simulink model "simulink_simulations"  (R2024a)
settings: Solver=VariableStepAuto  StartTime=0.0  StopTime=60  MaxStep=1e-2  RelTol=1e-3
values from neighbouring files (symbols this model uses):
  A = [0 1 0 0 ... (first row only)    [matlab_script.m]
  B = [0 0; 1/m 0; 0 0; 0 1/m]    [matlab_script.m]
  C = eye(4)    [matlab_script.m]
  D = zeros(4, 2)    [matlab_script.m]
  eta = 8e17    (= 8e+17)    [matlab_script.m]
  K = lqr(A, B, Q, R)    [matlab_script.m]
  K1 = 1    [matlab_script.m]
  K2 = 1    [matlab_script.m]
  m = 2e3    (= 2000)    [matlab_script.m]
  perturbation_standard_deviation = 9.6e7    (= 96000000)    [matlab_script.m]
  R_earth = 6.378e6    (= 6378000)    [matlab_script.m]
  x_eq = [r_ref; d_r_ref; theta_ref; d_theta_ref]    [matlab_script.m]
undefined symbols (not defined in the file or in its folder): Continuous, Time
libraries: ctrlSharedLib x2
settings Model: Creator=maxik  LastModifiedBy=maxik

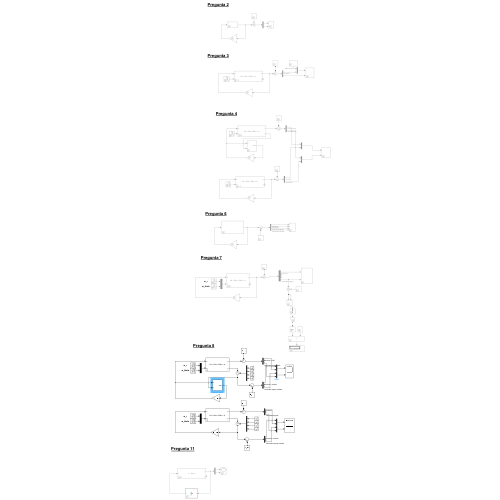
[thumbnail: Simulink's stored preview of the top-level diagram]
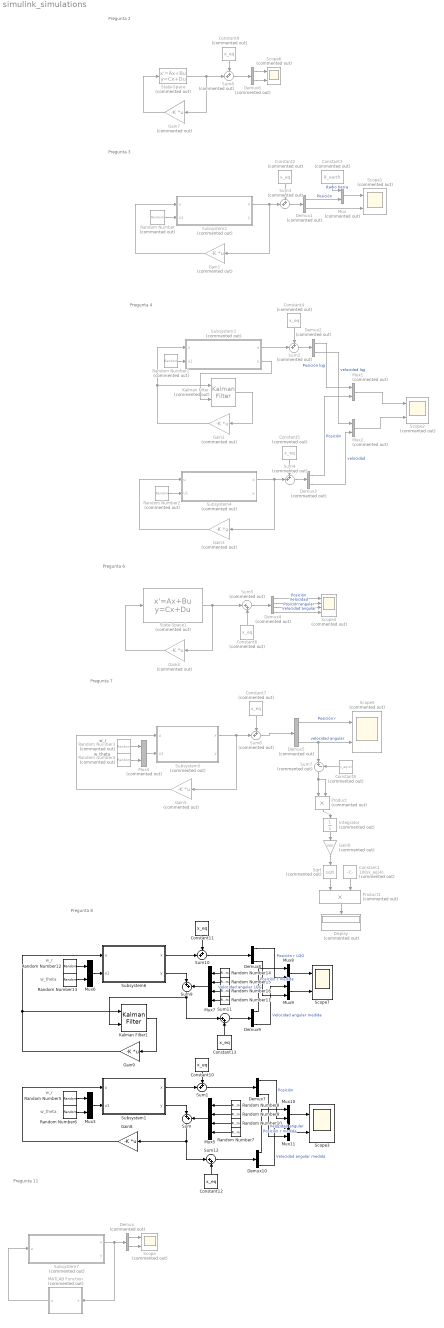
== system simulink_simulations ==
  note: Pregunta 8
  note: w_theta
  note: w_r
  note: Pregunta 2
  note: Pregunta 3
  note: Pregunta 4
  note: Pregunta 6
  note: Pregunta 7
  note: w_r
  note: w_theta
  note: w_theta
  note: w_r
  note: Pregunta 11
  Constant1 : Constant  Commented=on  Value=100/x_eq(4)
  Constant{10..13} (4 alike) : Constant  Value=x_eq
  Constant{2,4..7,9} (6 alike) : Constant  Commented=on  Value=x_eq
  Constant3 : Constant  Commented=on  Value=R_earth
  Constant8 : Constant  Commented=on  Value=x_eq(4)
  Demux{,1..3,6} (5 alike) : Demux  Commented=on  Outputs=2
  Demux{7..10} (4 alike) : Demux
  Demux4 : Demux  Commented=on
  Demux5 : Demux  Commented=on
  Display : Display  Commented=on
  Gain{1..5,7} (6 alike) : Gain  Commented=on  Gain=-K  Multiplication=Matrix(K*u) (u vector)
  Gain6 : Gain  Commented=on  Gain=1/60
  Gain8 : Gain  Gain=-K  Multiplication=Matrix(K*u) (u vector)
  Gain9 : Gain  Gain=-K  Multiplication=Matrix(K*u) (u vector)
  Integrator : Integrator  Commented=on
  Kalman Filter : ctrlSharedLib/Kalman Filter  Commented=on  TimeDomain=Continuous-Time  UseCurrentEstimator=on  ModelSource=Individual A, B, C, D matrices  ModelSourceVariable=ss(0.95,1,1,0,1)  A=A  B=B  C=C  D=D  NumberOfStates=1  NumberOfInputs=1  NumberOfOutputs=1  InitialEstimateSource=Dialog  X0=[0; 0]  P0=10  UseK=off  UseGH=on  NumberOfProcessNoiseInputs=1  G=[0; 1]  TimeInvariantG=on  H=[0; 0]  TimeInvariantH=on  Q=0 * (9.6e7)^2  TimeInvariantQ=on  R=1e-5 * eye(2)  TimeInvariantR=on  N=[0 0]  TimeInvariantN=on  AddInputPort=on  AddEnablePort=off  OutputEstimatedY=off  OutputP=off  Ts=-1
  Kalman Filter1 : ctrlSharedLib/Kalman Filter  TimeDomain=Continuous-Time  UseCurrentEstimator=on  ModelSource=Individual A, B, C, D matrices  ModelSourceVariable=ss(0.95,1,1,0,1)  A=A  B=B  C=C  D=D  NumberOfStates=1  NumberOfInputs=1  NumberOfOutputs=1  InitialEstimateSource=Dialog  X0=0  P0=10  UseK=off  UseGH=on  NumberOfProcessNoiseInputs=1  G=[0 0; 1 0; 0 0; 0 1]  TimeInvariantG=on  H=0  TimeInvariantH=on  Q="diag([(0.01*9.6e7)^2   (0.01*0.23)^2])"  TimeInvariantQ=on  R="diag([(1.6e5)^2  (1e4)^2  (1e-5)^2  (7.27e-6)^2])"  TimeInvariantR=on  N=0  TimeInvariantN=on  AddInputPort=on  AddEnablePort=off  OutputEstimatedY=off  OutputP=off  Ts=-1
  MATLAB Function : MATLAB Function  Commented=on  TreatAsAtomicUnit=on
  Mux{,1..2,4} (4 alike) : Mux  Commented=on  Inputs=2
  Mux{3,6,8..11} (6 alike) : Mux  Inputs=2
  Mux5 : Mux
  Mux7 : Mux
  Product : Product  Commented=on
  Product1 : Product  Commented=on
  Random Number : RandomNumber  Commented=on  Variance=perturbation_standard_deviation^2  Seed=25  SampleTime=1e-5
  Random Number1 : RandomNumber  Commented=on  Variance=(9.6e7)^2  Seed=25  SampleTime=1e-5
  Random Number10 : RandomNumber  Variance=(1e-5)^2  SampleTime=1e-5
  Random Number11 : RandomNumber  Variance=(7.27e-6)^2  SampleTime=1e-5
  Random Number12 : RandomNumber  Variance=(0.01 * 9.6e7)^2  Seed=25  SampleTime=1e-5
  Random Number13 : RandomNumber  Variance=(0.01 * 0.23)^2  Seed=25  SampleTime=1e-5
  Random Number14 : RandomNumber  Variance=(1.6e5)^2  SampleTime=1e-5
  Random Number15 : RandomNumber  Variance=(1e4)^2  SampleTime=1e-5
  Random Number16 : RandomNumber  Variance=(1e-5)^2  SampleTime=1e-5
  Random Number2 : RandomNumber  Commented=on  Variance=(9.6e7)^2  Seed=25  SampleTime=1e-5
  Random Number3 : RandomNumber  Commented=on  Variance=(0.01 * 9.6e7)^2  Seed=25  SampleTime=1e-5
  Random Number4 : RandomNumber  Commented=on  Variance=(0.23)^2  Seed=25  SampleTime=1e-5
  Random Number5 : RandomNumber  Variance=(0.01 * 9.6e7)^2  Seed=25  SampleTime=1e-5
  Random Number6 : RandomNumber  Variance=(0.01 * 0.23)^2  Seed=25  SampleTime=1e-5
  Random Number7 : RandomNumber  Variance=(7.27e-6)^2  SampleTime=1e-5
  Random Number8 : RandomNumber  Variance=(1.6e5)^2  SampleTime=1e-5
  Random Number9 : RandomNumber  Variance=(1e4)^2  SampleTime=1e-5
  Scope{,1..2,5..6} (5 alike) : Scope  Commented=on  NumInputPorts=2
  Scope3 : Scope  NumInputPorts=2
  Scope4 : Scope  Commented=on  NumInputPorts=4
  Scope7 : Scope  NumInputPorts=2
  Sqrt : Sqrt  Commented=on
  State-Space : StateSpace  Commented=on  A=A  B=B  C=C  D=D  InitialCondition=[1e6; -2e6]
  State-Space1 : StateSpace  Commented=on  A=A  B=B  C=C  D=D  InitialCondition=[-1e6; -1e6; 0; 0]
  Subsystem1 : Subsystem
      mask Display:
      | disp('\n\n\nΔẋ = AΔx + BΔu + w\n\n\n')
      | port_label('input', 1, 'u');
      | port_label('input', 2, 'w');
      | port_label('output', 1, 'x');
      | port_label('output', 2, 'y');
  Subsystem2 : Subsystem  Commented=on
      mask Display:
      | disp('\n\n\nΔẋ = AΔx + BΔu + w\n\n\n')
      | port_label('input', 1, 'u');
      | port_label('input', 2, 'w');
      | port_label('output', 1, 'x');
      | port_label('output', 2, 'y');
  Subsystem3 : Subsystem  Commented=on
      mask Display:
      | disp('\n\n\nΔẋ = AΔx + BΔu + w\n\n\n')
      | port_label('input', 1, 'u');
      | port_label('input', 2, 'w');
      | port_label('output', 1, 'x');
      | port_label('output', 2, 'y');
  Subsystem4 : Subsystem  Commented=on
      mask Display:
      | disp('\n\n\nΔẋ = AΔx + BΔu + w\n\n\n')
      | port_label('input', 1, 'u');
      | port_label('input', 2, 'w');
      | port_label('output', 1, 'x');
      | port_label('output', 2, 'y');
  Subsystem5 : Subsystem  Commented=on
      mask Display:
      | disp('\n\n\nΔẋ = AΔx + BΔu + w\n\n\n')
      | port_label('input', 1, 'u');
      | port_label('input', 2, 'w');
      | port_label('output', 1, 'x');
      | port_label('output', 2, 'y');
  Subsystem6 : Subsystem
      mask Display:
      | disp('\n\n\nΔẋ = AΔx + BΔu + w\n\n\n')
      | port_label('input', 1, 'u');
      | port_label('input', 2, 'w');
      | port_label('output', 1, 'x');
      | port_label('output', 2, 'y');
  Subsystem7 : Subsystem  Commented=on
      mask Display:
      | disp('\n\n\nẋ = f(x,u)\n\n\n')
      | port_label('input', 1, 'u');
      | port_label('output', 1, 'x');
      | port_label('output', 2, 'y');
  Sum{,9,11..12} (4 alike) : Sum  Inputs=|++
  Sum1 : Sum  Inputs=++|
  Sum10 : Sum  Inputs=++|
  Sum{2..4,6,8} (5 alike) : Sum  Commented=on  Inputs=++|
  Sum5 : Sum  Commented=on  Inputs=|++
  Sum7 : Sum  Commented=on  Inputs=|+-
  wires:
  Subsystem2/1(x) -> Gain1/1, Sum3/2
  Demux1/2 -> Scope1/2
  Random Number/1 -> Subsystem2/2(u1)
  Gain1/1 -> Subsystem2/1(u)
  Sum3/1 -> Demux1/1
  Constant2/1 -> Sum3/1
  Demux1/1 -> Mux/2  "Posición"
  Mux/1 -> Scope1/1
  Constant3/1 -> Mux/1  "Radio tierra"
  Gain2/1 -> Subsystem3/1(u), Kalman Filter/1
  Sum2/1 -> Demux2/1
  Subsystem3/1(x) -> Sum2/2
  Constant4/1 -> Sum2/1
  Random Number1/1 -> Subsystem3/2(u1)
  Subsystem3/2(y) -> Kalman Filter/2
  Kalman Filter/1 -> Gain2/1
  Sum4/1 -> Demux3/1
  Gain3/1 -> Subsystem4/1(u)
  Random Number2/1 -> Subsystem4/2(u1)
  Subsystem4/1(x) -> Gain3/1, Sum4/2
  Constant5/1 -> Sum4/1
  Demux2/1 -> Mux1/1  "Posición lqg"
  Demux3/1 -> Mux1/2  "Posición"
  Demux2/2 -> Mux2/1  "velocidad lqg"
  Demux3/2 -> Mux2/2  "velocidad"
  Mux2/1 -> Scope2/2
  Mux1/1 -> Scope2/1
  State-Space1/1 -> Sum5/1, Gain4/1
  Sum5/1 -> Demux4/1
  Gain4/1 -> State-Space1/1
  Constant6/1 -> Sum5/2
  Demux4/1 -> Scope4/1  "Posición"
  Demux4/4 -> Scope4/4  "Velocidad angular"
  Demux4/3 -> Scope4/3  "Posición angular"
  Demux4/2 -> Scope4/2  "Velocidad"
  Constant7/1 -> Sum6/1
  Gain5/1 -> Subsystem5/1(u)
  Subsystem5/1(x) -> Gain5/1, Sum6/2
  Sum6/1 -> Demux5/1
  Random Number3/1 -> Mux4/1
  Random Number4/1 -> Mux4/2
  Mux4/1 -> Subsystem5/2(u1)
  Demux5/1 -> Scope5/1  "Posición r"
  Demux5/4 -> Scope5/2, Sum7/1  "velocidad angular"
  Constant8/1 -> Sum7/2
  Sum7/1 -> Product/2, Product/1
  Product/1 -> Integrator/1
  Integrator/1 -> Gain6/1
  Gain6/1 -> Sqrt/1
  State-Space/1 -> Sum8/2, Gain7/1
  Gain7/1 -> State-Space/1
  Constant9/1 -> Sum8/1
  Demux6/2 -> Scope6/2
  Demux6/1 -> Scope6/1
  Sum8/1 -> Demux6/1
  Constant1/1 -> Product1/2
  Sqrt/1 -> Product1/1
  Product1/1 -> Display/1
  Mux3/1 -> Subsystem1/2(u1)
  Random Number5/1 -> Mux3/1
  Random Number6/1 -> Mux3/2
  Subsystem1/1(x) -> Sum1/2
  Constant10/1 -> Sum1/1
  Gain8/1 -> Subsystem1/1(u)
  Subsystem1/2(y) -> Sum/1
  Mux5/1 -> Sum/2
  Sum/1 -> Sum12/1, Gain8/1
  Random Number14/1 -> Mux7/1
  Random Number12/1 -> Mux6/1
  Random Number13/1 -> Mux6/2
  Mux6/1 -> Subsystem6/2(u1)
  Gain9/1 -> Subsystem6/1(u), Kalman Filter1/1
  Subsystem6/1(x) -> Sum10/2
  Random Number11/1 -> Mux7/4
  Constant11/1 -> Sum10/1
  Subsystem6/2(y) -> Sum9/1
  Mux7/1 -> Sum9/2
  Random Number15/1 -> Mux7/2
  Random Number16/1 -> Mux7/3
  Sum9/1 -> Sum11/1, Kalman Filter1/2
  Kalman Filter1/1 -> Gain9/1
  Sum1/1 -> Demux7/1
  Sum10/1 -> Demux8/1
  Subsystem7/1(x) -> Demux/1, MATLAB Function/1(x)
  MATLAB Function/1(u) -> Subsystem7/1(u)
  Demux/1 -> Scope/1
  Demux/2 -> Scope/2
  Random Number8/1 -> Mux5/1
  Random Number9/1 -> Mux5/2
  Random Number7/1 -> Mux5/4
  Random Number10/1 -> Mux5/3
  Mux8/1 -> Scope7/1
  Mux9/1 -> Scope7/2
  Mux10/1 -> Scope3/1
  Mux11/1 -> Scope3/2
  Sum11/1 -> Demux9/1
  Constant13/1 -> Sum11/2
  Constant12/1 -> Sum12/2
  Sum12/1 -> Demux10/1
  Demux7/1 -> Mux10/2  "Posición"
  Demux10/1 -> Mux10/1  "Posición r medida"
  Demux10/4 -> Mux11/1  "Velocidad angular medida"
  Demux7/4 -> Mux11/2  "Velocidad angular"
  Demux9/4 -> Mux9/1  "Velocidad angular medida"
  Demux8/4 -> Mux9/2  "Velocidad angular LQG"
  Demux9/1 -> Mux8/1  "Posición r medida"
  Demux8/1 -> Mux8/2  "Posición r LQG"

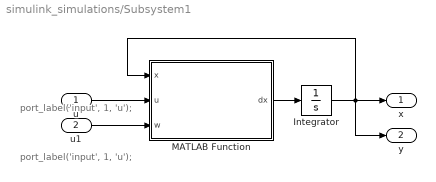
== system simulink_simulations/Subsystem1 ==
  note: port_label('input', 1, 'u');
  note: port_label('input', 1, 'u');
  u : Inport
  u1 : Inport  Port=2
  Integrator : Integrator  InitialCondition=zeros(4,1)
  MATLAB Function : MATLAB Function  TreatAsAtomicUnit=on
  x : Outport
  y : Outport  Port=2
  wires:
  MATLAB Function/1(dx) -> Integrator/1
  Integrator/1 -> y/1, x/1, MATLAB Function/1(x)
  u/1 -> MATLAB Function/2(u)
  u1/1 -> MATLAB Function/3(w)

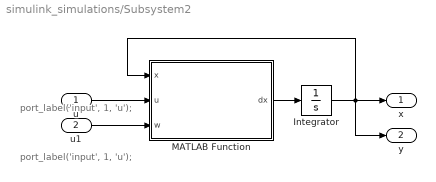
== system simulink_simulations/Subsystem2 ==
  note: port_label('input', 1, 'u');
  note: port_label('input', 1, 'u');
  u : Inport
  u1 : Inport  Port=2
  Integrator : Integrator  InitialCondition=zeros(2,1)
  MATLAB Function : MATLAB Function  TreatAsAtomicUnit=on
  x : Outport
  y : Outport  Port=2
  wires:
  MATLAB Function/1(dx) -> Integrator/1
  Integrator/1 -> y/1, x/1, MATLAB Function/1(x)
  u/1 -> MATLAB Function/2(u)
  u1/1 -> MATLAB Function/3(w)

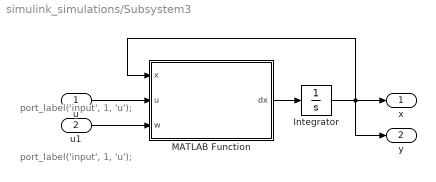
== system simulink_simulations/Subsystem3 ==
  note: port_label('input', 1, 'u');
  note: port_label('input', 1, 'u');
  u : Inport
  u1 : Inport  Port=2
  Integrator : Integrator  InitialCondition=zeros(2,1)
  MATLAB Function : MATLAB Function  TreatAsAtomicUnit=on
  x : Outport
  y : Outport  Port=2
  wires:
  MATLAB Function/1(dx) -> Integrator/1
  Integrator/1 -> y/1, x/1, MATLAB Function/1(x)
  u/1 -> MATLAB Function/2(u)
  u1/1 -> MATLAB Function/3(w)

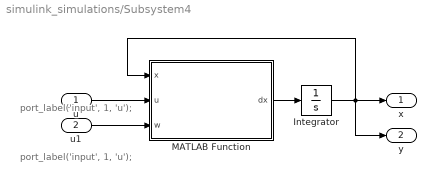
== system simulink_simulations/Subsystem4 ==
  note: port_label('input', 1, 'u');
  note: port_label('input', 1, 'u');
  u : Inport
  u1 : Inport  Port=2
  Integrator : Integrator  InitialCondition=zeros(2,1)
  MATLAB Function : MATLAB Function  TreatAsAtomicUnit=on
  x : Outport
  y : Outport  Port=2
  wires:
  MATLAB Function/1(dx) -> Integrator/1
  Integrator/1 -> y/1, x/1, MATLAB Function/1(x)
  u/1 -> MATLAB Function/2(u)
  u1/1 -> MATLAB Function/3(w)

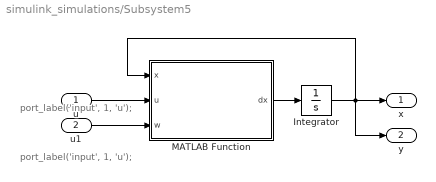
== system simulink_simulations/Subsystem5 ==
  note: port_label('input', 1, 'u');
  note: port_label('input', 1, 'u');
  u : Inport
  u1 : Inport  Port=2
  Integrator : Integrator  InitialCondition=zeros(4,1)
  MATLAB Function : MATLAB Function  TreatAsAtomicUnit=on
  x : Outport
  y : Outport  Port=2
  wires:
  MATLAB Function/1(dx) -> Integrator/1
  Integrator/1 -> y/1, x/1, MATLAB Function/1(x)
  u/1 -> MATLAB Function/2(u)
  u1/1 -> MATLAB Function/3(w)

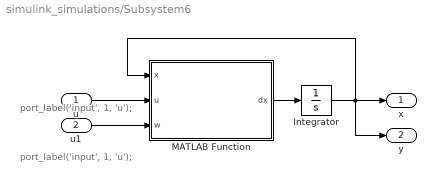
== system simulink_simulations/Subsystem6 ==
  note: port_label('input', 1, 'u');
  note: port_label('input', 1, 'u');
  u : Inport
  u1 : Inport  Port=2
  Integrator : Integrator  InitialCondition=zeros(4,1)
  MATLAB Function : MATLAB Function  TreatAsAtomicUnit=on
  x : Outport
  y : Outport  Port=2
  wires:
  MATLAB Function/1(dx) -> Integrator/1
  Integrator/1 -> y/1, x/1, MATLAB Function/1(x)
  u/1 -> MATLAB Function/2(u)
  u1/1 -> MATLAB Function/3(w)

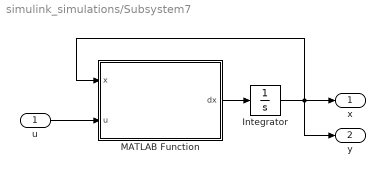
== system simulink_simulations/Subsystem7 ==
  u : Inport
  Integrator : Integrator  InitialCondition=[2; 0]
  MATLAB Function : MATLAB Function  TreatAsAtomicUnit=on
  x : Outport
  y : Outport  Port=2
  wires:
  MATLAB Function/1(dx) -> Integrator/1
  Integrator/1 -> y/1, x/1, MATLAB Function/1(x)
  u/1 -> MATLAB Function/2(u)

== matlab function simulink_simulations/MATLAB Function ==
  data: x input; u output; m parameter; eta parameter; x_eq parameter; K1 parameter; K2 parameter
function u = fcn(x, m, eta, x_eq, K1, K2)
    
    u = m * ((-K1 * x(2)) - (x(1) - x_eq(1)) + (eta/x(1)^2) -K2 * (x(2) + K1 * (x(1) - x_eq(1))));

== matlab function simulink_simulations/Subsystem1/MATLAB Function ==
  data: x input; u input; w input; dx output; A parameter; B parameter
function dx = fcn(x, u, w, A, B)

    dx = A * x + B * u + [0; w(1); 0; w(2)];


end

== matlab function simulink_simulations/Subsystem2/MATLAB Function ==
  data: x input; u input; w input; dx output; A parameter; B parameter; x_eq parameter; R_earth parameter
function dx = fcn(x, u, w, A, B, x_eq, R_earth)

    if x(1) >= -(x_eq(1) - R_earth)
        dx = A * x + B * u + [0; w];

    else
        dx = zeros(2,1);

    end

end

== matlab function simulink_simulations/Subsystem3/MATLAB Function ==
  data: x input; u input; w input; dx output; A parameter; B parameter; R_earth parameter; x_eq parameter
function dx = fcn(x, u, w, A, B, R_earth, x_eq)


    if x(1) >= -(x_eq(1) - R_earth)
        dx = A * x + B * u + [0; w];

    else
        dx = zeros(2,1);

    end

end

== matlab function simulink_simulations/Subsystem4/MATLAB Function ==
  data: x input; u input; w input; dx output; A parameter; B parameter; x_eq parameter; R_earth parameter
function dx = fcn(x, u, w, A, B, x_eq, R_earth)

    if x(1) >= -(x_eq(1) - R_earth)
        dx = A * x + B * u + [0; w];

    else
        dx = zeros(2,1);

    end

end

== matlab function simulink_simulations/Subsystem5/MATLAB Function ==
  data: x input; u input; w input; dx output; A parameter; B parameter
function dx = fcn(x, u, w, A, B)

    dx = A * x + B * u + [0; w(1); 0; w(2)];


end

== matlab function simulink_simulations/Subsystem6/MATLAB Function ==
  data: x input; u input; w input; dx output; A parameter; B parameter
function dx = fcn(x, u, w, A, B)

    dx = A * x + B * u + [0; w(1); 0; w(2)];


end

== matlab function simulink_simulations/Subsystem7/MATLAB Function ==
  data: x input; u input; dx output; eta parameter; m parameter
function dx = fcn(x, u, eta, m)

    dx = zeros(2,1);
    dx(1) = x(2);
    dx(2) = -(eta/x(1)^2) + (u/m);

end
